simulink subsystem "Plant"  (R2024b)
settings: Solver=VariableStepAuto  StartTime=0.0  StopTime=10.0  RelTol=1e-3
values from neighbouring files (symbols this model uses):
  Ar = 0.0181458391671    [barrowaman.mat]
  CndNi_canard = (N_canard * (c1_canard + c2_canard + c3_canard))/(Ar * (Lr))    [Barrowman_Equations.m]    (also in barrowaman.mat = 1.83025622565)
  Cnfdelta_canard = N_canard * Y_canard / span_canard    [Barrowman_Equations.m]    (also in barrowaman.mat = 5.8)
  Lr = 0.152    [barrowaman.mat]
  Mdot = [-2.06885767428 -2.65545019236 -3.15692906995 -3.53463604631 -3.77514336449 -3.88832803946 -3.9029455228 -3.85572128709 -3.78250824721 -3.71051505737 -3.65407665098 -3.61686646614 ... (1300 elements, 1300x1)]    [barrowaman.mat]
  rail_angle = 0.0872664625997    [barrowaman.mat]
  sim_time = [0.01 0.02 0.03 0.04 0.05 0.06 0.07 0.08 0.09 0.1 0.11 0.12 ... (1300 elements, 1300x1)]    [barrowaman.mat]
  Y = rt + (span/3) * yparcial    [Barrowman_Equations.m]    (also in barrowaman.mat = 0.163464458247)
undefined symbols (not defined in the file or in its folder): Cndomega
libraries: shared6dof x1
settings Model: Creator=joedo  LastModifiedBy=joedo

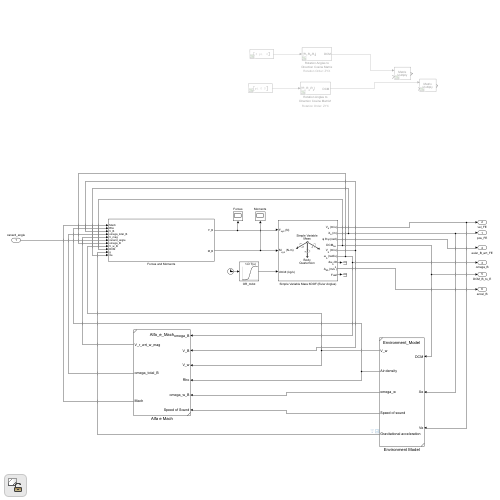
[thumbnail: Simulink's stored preview of the top-level diagram]
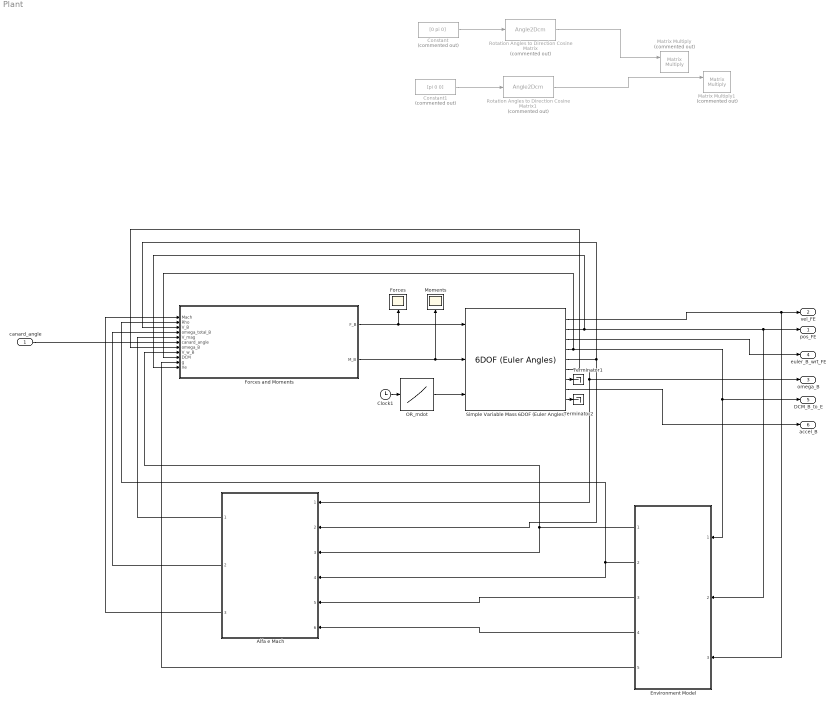
== system Plant ==
  canard_angle : Inport
  Alfa e Mach : Subsystem  ReferencedSubsystem=Alfa_e_Mach
  Clock1 : Clock
  Constant : Constant  Commented=on  Value=[0 pi 0]
  Constant1 : Constant  Commented=on  Value=[pi 0 0]
  Environment Model : Subsystem  ReferencedSubsystem=Environment_Model
  Forces : Scope
  "Forces and Moments " : Subsystem
  Matrix Multiply : Product  Commented=on  Multiplication=Matrix(*)
  Matrix Multiply1 : Product  Commented=on  Multiplication=Matrix(*)
  Moments : Scope
  OR_mdot : Lookup_n-D  NumberOfTableDimensions=1  BreakpointsForDimension1=sim_time  Table=Mdot  InternalRulePriority=Speed  RndMeth=Simplest
  Rotation Angles to Direction Cosine Matrix : Angle2Dcm  Commented=on
      settings: AttributesFormatString=Rotation Order: %<rotationOrder>
  Rotation Angles to Direction Cosine Matrix1 : Angle2Dcm  Commented=on
      settings: AttributesFormatString=Rotation Order: %<rotationOrder>
  Simple Variable Mass 6DOF (Euler Angles) : shared6dof/6DOF (Euler Angles)  units=Metric (MKS)  mtype=Simple Variable  rep=Quaternion  xme_0=[0 0 0]  Vm_0=[0 0 0]  eul_0=[0 pi/2 + rail_angle 0]  pm_0=[0 0 0]  mass_0=total_mass_0  mass_e=total_mass_d  mass_f=total_mass_0  inertia=eye(3)  inertia_e=I_d  inertia_f=I_0  k_quat=1.0  vre_flag=off  abi_flag=off  aMode=aMode  xme_statename=''  Vm_statename=''  eul_statename=''  quat_statename=''  pm_statename=''  mass_statename=''
  Terminator1 : Terminator
  Terminator2 : Terminator
  pos_FE : Outport
  vel_FE : Outport  Port=2
  omega_B : Outport  Port=3
  euler_B_wrt_FE : Outport  Port=4
  DCM_B_to_E : Outport  Port=5
  accel_B : Outport  Port=6
  wires:
  "Forces and Moments "/1(F_B) -> Simple Variable Mass 6DOF (Euler Angles)/1, Forces/1
  Alfa e Mach/1 -> "Forces and Moments "/5("V_mag ")
  canard_angle/1 -> "Forces and Moments "/6(canard_angle)
  Simple Variable Mass 6DOF (Euler Angles)/4 -> "Forces and Moments "/9(DCM), DCM_B_to_E/1, Environment Model/1
  Simple Variable Mass 6DOF (Euler Angles)/6 -> "Forces and Moments "/7(omega_B), omega_B/1, Alfa e Mach/1
  Simple Variable Mass 6DOF (Euler Angles)/5 -> "Forces and Moments "/3(V_B), Alfa e Mach/2
  Environment Model/1 -> Alfa e Mach/3, "Forces and Moments "/8(V_w_B)
  Alfa e Mach/2 -> "Forces and Moments "/4(omega_total_B)
  Environment Model/3 -> Alfa e Mach/5
  Environment Model/2 -> Alfa e Mach/4, "Forces and Moments "/2(Rho)
  "Forces and Moments "/2(M_B) -> Simple Variable Mass 6DOF (Euler Angles)/2, Moments/1
  Environment Model/4 -> Alfa e Mach/6
  Simple Variable Mass 6DOF (Euler Angles)/2 -> pos_FE/1, Environment Model/2, "Forces and Moments "/11(Xe)
  Alfa e Mach/3 -> "Forces and Moments "/1(Mach)
  Simple Variable Mass 6DOF (Euler Angles)/7 -> Terminator1/1
  OR_mdot/1 -> Simple Variable Mass 6DOF (Euler Angles)/3
  Simple Variable Mass 6DOF (Euler Angles)/8 -> accel_B/1
  Simple Variable Mass 6DOF (Euler Angles)/9 -> Terminator2/1
  Environment Model/5 -> "Forces and Moments "/10(g)
  Constant1/1 -> Rotation Angles to Direction Cosine Matrix1/1
  Constant/1 -> Rotation Angles to Direction Cosine Matrix/1
  Rotation Angles to Direction Cosine Matrix1/1 -> Matrix Multiply1/1
  Rotation Angles to Direction Cosine Matrix/1 -> Matrix Multiply/1
  Clock1/1 -> OR_mdot/1
  Simple Variable Mass 6DOF (Euler Angles)/1 -> vel_FE/1, Environment Model/3
  Simple Variable Mass 6DOF (Euler Angles)/3 -> euler_B_wrt_FE/1

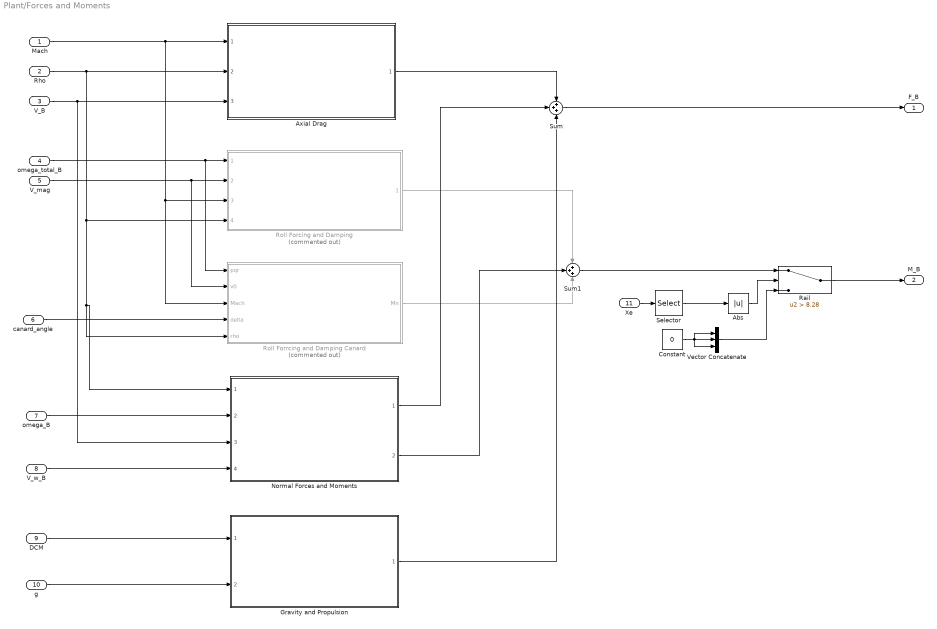
== system Plant/Forces and Moments  ==
  Mach : Inport
  Rho : Inport  Port=2
  V_B : Inport  Port=3
  omega_total_B : Inport  Port=4
  "V_mag " : Inport  Port=5
  canard_angle : Inport  Port=6
  omega_B : Inport  Port=7
  V_w_B : Inport  Port=8
  DCM : Inport  Port=9
  g : Inport  Port=10
  Xe : Inport  Port=11
  Abs : Abs  SaturateOnIntegerOverflow=off
  Axial Drag : Subsystem  ReferencedSubsystem=Axial_Drag
  Constant : Constant  Value=0
  Gravity and Propulsion : Subsystem  ReferencedSubsystem=Gravity_and_Propulsion
  Normal Forces and Moments : Subsystem  ReferencedSubsystem=Normal_Forces_and_Moments
  Rail : Switch  Criteria=u2 > Threshold  Threshold=8.28  SaturateOnIntegerOverflow=off  InputSameDT=off
  Roll Forcing and Damping : Subsystem  Commented=on  ReferencedSubsystem=Roll_Forcing_and_Damping
  Roll Forrcing and Damping Canard : Subsystem  Commented=on
  Selector : Selector  InputPortWidth=3  IndexOptions=Index vector (dialog)  Indices=[3]  OutputSizes=1
  Sum : Sum  Inputs=3
  Sum1 : Sum  Inputs=3
  Vector Concatenate : Concatenate  NumInputs=3
  F_B : Outport  VectorParamsAs1DForOutWhenUnconnected=off
  M_B : Outport  Port=2  VectorParamsAs1DForOutWhenUnconnected=off
  wires:
  Vector Concatenate/1 -> Rail/3
  Constant/1 -> Vector Concatenate/1, Vector Concatenate/3, Vector Concatenate/2
  Abs/1 -> Rail/2
  Selector/1 -> Abs/1
  Xe/1 -> Selector/1
  Rail/1 -> M_B/1
  g/1 -> Gravity and Propulsion/2
  Roll Forcing and Damping/1 -> Sum1/1
  Roll Forrcing and Damping Canard/1(Mn) -> Sum1/3
  canard_angle/1 -> Roll Forrcing and Damping Canard/4(delta)
  Normal Forces and Moments/2 -> Sum1/2
  Normal Forces and Moments/1 -> Sum/2
  V_w_B/1 -> Normal Forces and Moments/4
  V_B/1 -> Axial Drag/3, Normal Forces and Moments/3
  omega_B/1 -> Normal Forces and Moments/2
  Sum1/1 -> Rail/1
  Axial Drag/1 -> Sum/1
  DCM/1 -> Gravity and Propulsion/1
  Gravity and Propulsion/1 -> Sum/3
  Sum/1 -> F_B/1
  Rho/1 -> Axial Drag/2, Roll Forcing and Damping/4, Normal Forces and Moments/1, Roll Forrcing and Damping Canard/5(rho)
  "V_mag "/1 -> Roll Forcing and Damping/2, Roll Forrcing and Damping Canard/2("v0 ")
  omega_total_B/1 -> Roll Forrcing and Damping Canard/1(pqr), Roll Forcing and Damping/1
  Mach/1 -> Axial Drag/1, Roll Forcing and Damping/3, Roll Forrcing and Damping Canard/3("Mach ")

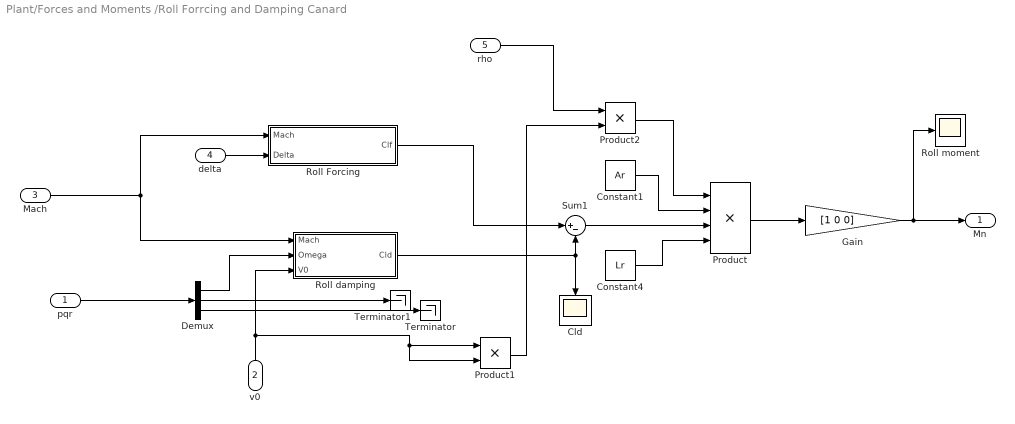
== system Plant/Forces and Moments /Roll Forrcing and Damping Canard ==
  pqr : Inport
  "v0 " : Inport  Port=2
  "Mach " : Inport  Port=3
  delta : Inport  Port=4
  rho : Inport  Port=5
  Cld : Scope
  Constant1 : Constant  Value=Ar
  Constant4 : Constant  Value=Lr
  Demux : Demux  Outputs=3
  Gain : Gain  Gain=[1 0 0]
  Product : Product  Inputs=4
  Product1 : Product
  Product2 : Product
  Roll Forcing : Subsystem
  "Roll damping " : Subsystem
  Roll moment : Scope
  Sum1 : Sum  Inputs=|+-
  Terminator : Terminator
  Terminator1 : Terminator
  Mn : Outport  VectorParamsAs1DForOutWhenUnconnected=off
  wires:
  Product/1 -> Gain/1
  delta/1 -> Roll Forcing/2(Delta)
  pqr/1 -> Demux/1
  Demux/1 -> "Roll damping "/2(Omega)
  Demux/2 -> Terminator1/1
  Gain/1 -> Roll moment/1, Mn/1
  Constant4/1 -> Product/4
  Product1/1 -> Product2/2
  "Mach "/1 -> "Roll damping "/1("Mach "), Roll Forcing/1(Mach)
  Demux/3 -> Terminator/1
  "Roll damping "/1(Cld) -> Sum1/2, Cld/1
  Sum1/1 -> Product/3
  rho/1 -> Product2/1
  Product2/1 -> Product/1
  "v0 "/1 -> Product1/1, Product1/2, "Roll damping "/3(V0)
  Constant1/1 -> Product/2
  Roll Forcing/1(Clf) -> Sum1/1

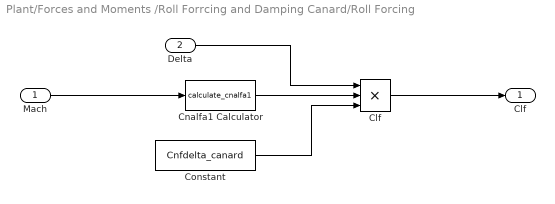
== system Plant/Forces and Moments /Roll Forrcing and Damping Canard/Roll Forcing ==
  Mach : Inport
  Delta : Inport  Port=2
  "Clf " : Product  Inputs=***
  "Cnalfa1 Calculator " : MATLABFcn  MATLABFcn=calculate_cnalfa1
  Constant : Constant  Value=Cnfdelta_canard
  Clf : Outport
  wires:
  Mach/1 -> "Cnalfa1 Calculator "/1
  "Clf "/1 -> Clf/1
  Constant/1 -> "Clf "/3
  "Cnalfa1 Calculator "/1 -> "Clf "/2
  Delta/1 -> "Clf "/1

== system Plant/Forces and Moments /Roll Forrcing and Damping Canard/Roll damping  ==
  "Mach " : Inport
  Omega : Inport  Port=2
  V0 : Inport  Port=3
  Damping Subsônico : Subsystem
  Supersônico : Subsystem  Commented=on
  Cld : Outport  VectorParamsAs1DForOutWhenUnconnected=off
  wires:
  Damping Subsônico/1(Cld) -> Cld/1
  V0/1 -> Damping Subsônico/3("v0 "), Supersônico/3(V0 2)
  Omega/1 -> Supersônico/2(Omega 1), Damping Subsônico/2(Omega)
  "Mach "/1 -> Supersônico/1("Mach "), Damping Subsônico/1("Mach ")

== system Plant/Forces and Moments /Roll Forrcing and Damping Canard/Roll damping /Damping Subsônico ==
  note: Cld= Cld(ni) * omega / v0
  "Mach " : Inport
  Omega : Inport  Port=2
  "v0 " : Inport  Port=3
  "CndNi " : Subsystem
  "Multiply " : Product  Inputs=**/
  Cld : Outport
  wires:
  Omega/1 -> "Multiply "/2
  "v0 "/1 -> "Multiply "/3
  "Mach "/1 -> "CndNi "/1("Mach ")
  "CndNi "/1(CndNi) -> "Multiply "/1
  "Multiply "/1 -> Cld/1

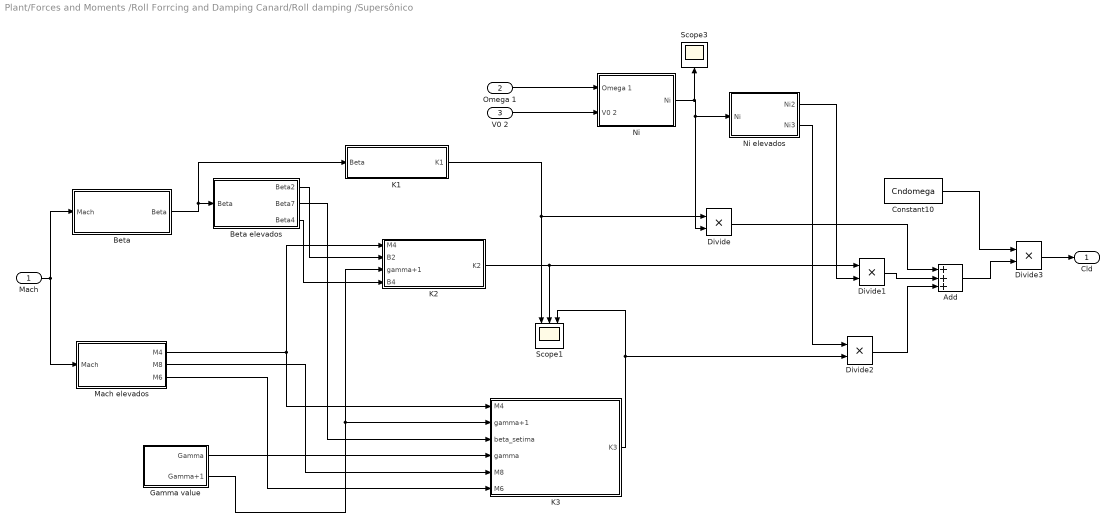
== system Plant/Forces and Moments /Roll Forrcing and Damping Canard/Roll damping /Supersônico ==
  "Mach " : Inport
  Omega 1 : Inport  Port=2
  V0 2 : Inport  Port=3
  Add : Sum  Inputs=+++
  Beta : Subsystem
  Beta elevados : Subsystem
  Constant10 : Constant  Value=Cndomega
  Divide{,1..3} (4 alike) : Product  Inputs=**
  Gamma value : Subsystem
  K1 : Subsystem
  K2 : Subsystem
  K3 : Subsystem
  Mach elevados : Subsystem
  Ni : Subsystem
  Ni elevados : Subsystem
  Scope1 : Scope  NumInputPorts=3
  Scope3 : Scope
  Cld : Outport  VectorParamsAs1DForOutWhenUnconnected=off
  wires:
  Beta elevados/3(Beta4) -> K2/4(B4)
  Beta elevados/1(Beta2) -> K2/2(B2)
  Beta elevados/2(Beta7) -> K3/3(beta_setima)
  K3/1(K3) -> Divide2/2, Scope1/3
  K1/1(K1) -> Scope1/1, Divide/1
  Add/1 -> Divide3/2
  Divide2/1 -> Add/3
  Mach elevados/2(M8) -> K3/5(M8)
  Mach elevados/1(M4) -> K3/1(M4), K2/1(" M4")
  Ni elevados/2(Ni3) -> Divide2/1
  Mach elevados/3(M6) -> K3/6(M6)
  Ni elevados/1(Ni2) -> Divide1/2
  Divide/1 -> Add/1
  Gamma value/1(Gamma) -> K3/4(gamma)
  Beta/1(Beta) -> K1/1(Beta), Beta elevados/1(Beta)
  Constant10/1 -> Divide3/1
  Divide1/1 -> Add/2
  V0 2/1 -> Ni/2(V0 2)
  K2/1(K2) -> Divide1/1, Scope1/2
  "Mach "/1 -> Beta/1(Mach), Mach elevados/1(Mach)
  Gamma value/2(Gamma+1) -> K3/2(gamma+1), K2/3(gamma+1)
  Omega 1/1 -> Ni/1(Omega 1)
  Divide3/1 -> Cld/1
  Ni/1(Ni) -> Scope3/1, Divide/2, Ni elevados/1(Ni)

== system Plant/Forces and Moments /Roll Forrcing and Damping Canard/Roll damping /Damping Subsônico/CndNi  ==
  "Mach " : Inport
  Cnalfa0 : Subsystem
  Constant2 : Constant  Value=CndNi_canard
  Product1 : Product
  CndNi : Outport  VectorParamsAs1DForOutWhenUnconnected=off
  wires:
  Cnalfa0/1("2pi / beta ") -> Product1/1
  "Mach "/1 -> Cnalfa0/1(Mach)
  Product1/1 -> CndNi/1
  Constant2/1 -> Product1/2

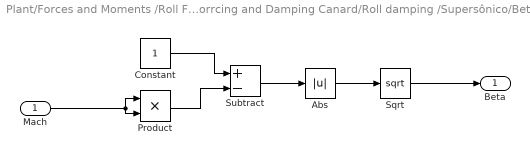
== system Plant/Forces and Moments /Roll Forrcing and Damping Canard/Roll damping /Supersônico/Beta ==
  Mach : Inport
  Abs : Abs  SaturateOnIntegerOverflow=off
  Constant : Constant
  Product : Product
  Sqrt : Sqrt
  Subtract : Sum  Inputs=+-
  Beta : Outport
  wires:
  Sqrt/1 -> Beta/1
  Abs/1 -> Sqrt/1
  Constant/1 -> Subtract/1
  Subtract/1 -> Abs/1
  Mach/1 -> Product/2, Product/1
  Product/1 -> Subtract/2

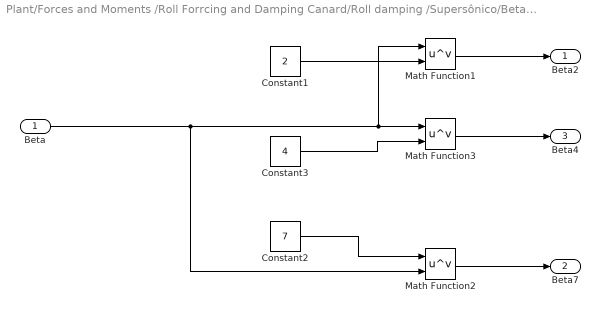
== system Plant/Forces and Moments /Roll Forrcing and Damping Canard/Roll damping /Supersônico/Beta elevados ==
  Beta : Inport
  Constant1 : Constant  Value=2
  Constant2 : Constant  Value=7
  Constant3 : Constant  Value=4
  Math Function1 : Math  Operator=pow
  Math Function2 : Math  Operator=pow
  Math Function3 : Math  Operator=pow
  Beta2 : Outport
  Beta7 : Outport  Port=2
  Beta4 : Outport  Port=3
  wires:
  Math Function3/1 -> Beta4/1
  Constant3/1 -> Math Function3/2
  Constant1/1 -> Math Function1/2
  Constant2/1 -> Math Function2/1
  Math Function1/1 -> Beta2/1
  Math Function2/1 -> Beta7/1
  Beta/1 -> Math Function2/2, Math Function1/1, Math Function3/1

== system Plant/Forces and Moments /Roll Forrcing and Damping Canard/Roll damping /Supersônico/Gamma value ==
  Constant4 : Constant  Value=1.4
  Constant5 : Constant
  Sum : Sum  Inputs=|++
  Gamma : Outport
  Gamma+1 : Outport  Port=2
  wires:
  Sum/1 -> Gamma+1/1
  Constant4/1 -> Sum/1, Gamma/1
  Constant5/1 -> Sum/2

== system Plant/Forces and Moments /Roll Forrcing and Damping Canard/Roll damping /Supersônico/K1 ==
  Beta : Inport
  Constant3 : Constant  Value=2
  Divide : Product  Inputs=*/
  K1 : Outport
  wires:
  Beta/1 -> Divide/2
  Divide/1 -> K1/1
  Constant3/1 -> Divide/1

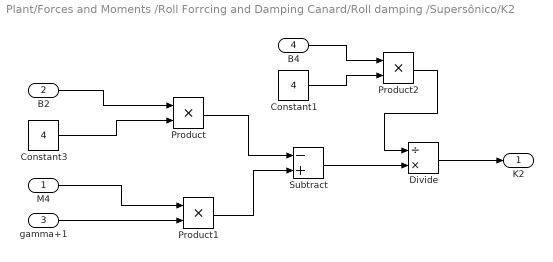
== system Plant/Forces and Moments /Roll Forrcing and Damping Canard/Roll damping /Supersônico/K2 ==
  " M4" : Inport
  B2 : Inport  Port=2
  gamma+1 : Inport  Port=3
  B4 : Inport  Port=4
  Constant1 : Constant  Value=4
  Constant3 : Constant  Value=4
  Divide : Product  Inputs=/*
  Product : Product
  Product1 : Product
  Product2 : Product
  Subtract : Sum  Inputs=-+
  K2 : Outport
  wires:
  Product2/1 -> Divide/1
  B4/1 -> Product2/1
  Constant1/1 -> Product2/2
  Subtract/1 -> Divide/2
  Product/1 -> Subtract/1
  Product1/1 -> Subtract/2
  B2/1 -> Product/1
  gamma+1/1 -> Product1/2
  " M4"/1 -> Product1/1
  Constant3/1 -> Product/2
  Divide/1 -> K2/1

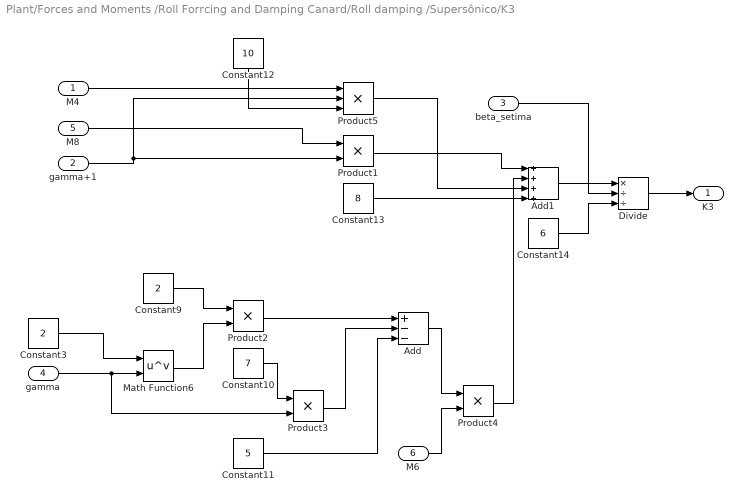
== system Plant/Forces and Moments /Roll Forrcing and Damping Canard/Roll damping /Supersônico/K3 ==
  M4 : Inport
  gamma+1 : Inport  Port=2
  beta_setima : Inport  Port=3
  gamma : Inport  Port=4
  M8 : Inport  Port=5
  M6 : Inport  Port=6
  Add : Sum  Inputs=+--
  Add1 : Sum  Inputs=++++
  Constant10 : Constant  Value=7
  Constant11 : Constant  Value=5
  Constant12 : Constant  Value=10
  Constant13 : Constant  Value=8
  Constant14 : Constant  Value=6
  Constant3 : Constant  Value=2
  Constant9 : Constant  Value=2
  Divide : Product  Inputs=*//
  Math Function6 : Math  Operator=pow
  Product{1..4} (4 alike) : Product
  Product5 : Product  Inputs=3
  K3 : Outport
  wires:
  M8/1 -> Product1/1
  M4/1 -> Product5/1
  M6/1 -> Product4/2
  Add1/1 -> Divide/1
  Product5/1 -> Add1/3
  Constant9/1 -> Product2/1
  Product3/1 -> Add/2
  Constant13/1 -> Add1/4
  Constant14/1 -> Divide/3
  Constant10/1 -> Product3/1
  Constant11/1 -> Add/3
  Constant12/1 -> Product5/3
  Math Function6/1 -> Product2/2
  Product1/1 -> Add1/1
  gamma/1 -> Math Function6/2, Product3/2
  gamma+1/1 -> Product1/2, Product5/2
  Divide/1 -> K3/1
  Constant3/1 -> Math Function6/1
  Add/1 -> Product4/1
  Product4/1 -> Add1/2
  beta_setima/1 -> Divide/2
  Product2/1 -> Add/1

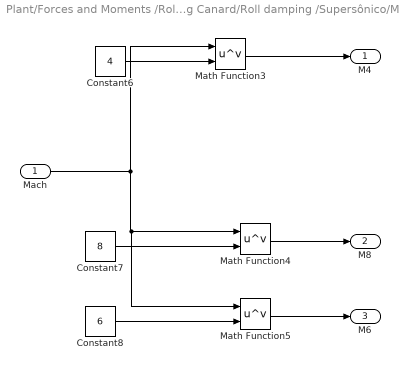
== system Plant/Forces and Moments /Roll Forrcing and Damping Canard/Roll damping /Supersônico/Mach elevados ==
  Mach : Inport
  Constant6 : Constant  Value=4
  Constant7 : Constant  Value=8
  Constant8 : Constant  Value=6
  Math Function3 : Math  Operator=pow
  Math Function4 : Math  Operator=pow
  Math Function5 : Math  Operator=pow
  M4 : Outport
  M8 : Outport  Port=2
  M6 : Outport  Port=3
  wires:
  Constant6/1 -> Math Function3/2
  Math Function5/1 -> M6/1
  Math Function4/1 -> M8/1
  Math Function3/1 -> M4/1
  Mach/1 -> Math Function3/1, Math Function4/1, Math Function5/1
  Constant8/1 -> Math Function5/2
  Constant7/1 -> Math Function4/2

== system Plant/Forces and Moments /Roll Forrcing and Damping Canard/Roll damping /Supersônico/Ni ==
  Omega 1 : Inport
  V0 2 : Inport  Port=2
  Atan : Trigonometry  Operator=atan
  Constant3 : Constant  Value=Y
  Divide : Product  Inputs=**/
  Ni : Outport
  wires:
  Atan/1 -> Ni/1
  Divide/1 -> Atan/1
  V0 2/1 -> Divide/3
  Constant3/1 -> Divide/1
  Omega 1/1 -> Divide/2

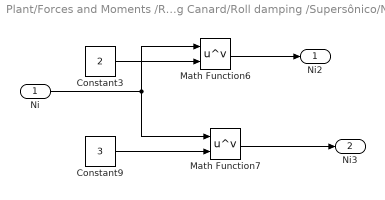
== system Plant/Forces and Moments /Roll Forrcing and Damping Canard/Roll damping /Supersônico/Ni elevados ==
  Ni : Inport
  Constant3 : Constant  Value=2
  Constant9 : Constant  Value=3
  Math Function6 : Math  Operator=pow
  Math Function7 : Math  Operator=pow
  Ni2 : Outport
  Ni3 : Outport  Port=2
  wires:
  Constant9/1 -> Math Function7/2
  Math Function7/1 -> Ni3/1
  Constant3/1 -> Math Function6/2
  Ni/1 -> Math Function6/1, Math Function7/1
  Math Function6/1 -> Ni2/1

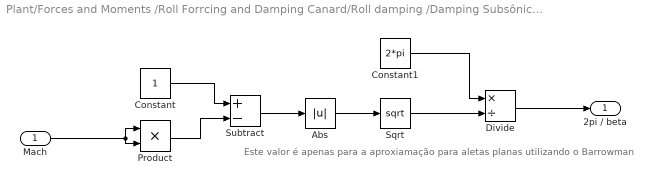
== system Plant/Forces and Moments /Roll Forrcing and Damping Canard/Roll damping /Damping Subsônico/CndNi /Cnalfa0 ==
  note: Este valor é apenas para a aproxiamação para aletas planas utilizando o Barrowman
  Mach : Inport
  Abs : Abs  SaturateOnIntegerOverflow=off
  Constant : Constant
  Constant1 : Constant  Value=2*pi
  Divide : Product  Inputs=*/
  Product : Product
  Sqrt : Sqrt
  Subtract : Sum  Inputs=+-
  "2pi / beta " : Outport
  wires:
  Divide/1 -> "2pi / beta "/1
  Subtract/1 -> Abs/1
  Constant/1 -> Subtract/1
  Mach/1 -> Product/2, Product/1
  Constant1/1 -> Divide/1
  Abs/1 -> Sqrt/1
  Product/1 -> Subtract/2
  Sqrt/1 -> Divide/2
